simulink model "sampleModel1545"  (R2023a)
settings: Solver=VariableStepAuto  StartTime=0.0  StopTime=10.0  RelTol=1e-3
libraries: hdlsllib x5, simulink x1
settings Model: Creator=user1  LastModifiedBy=user1

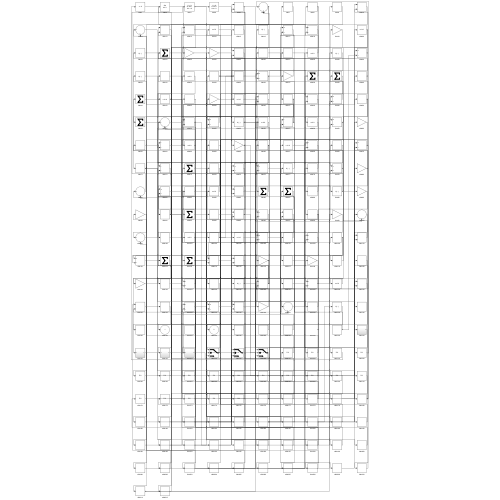
[thumbnail: Simulink's stored preview of the top-level diagram]
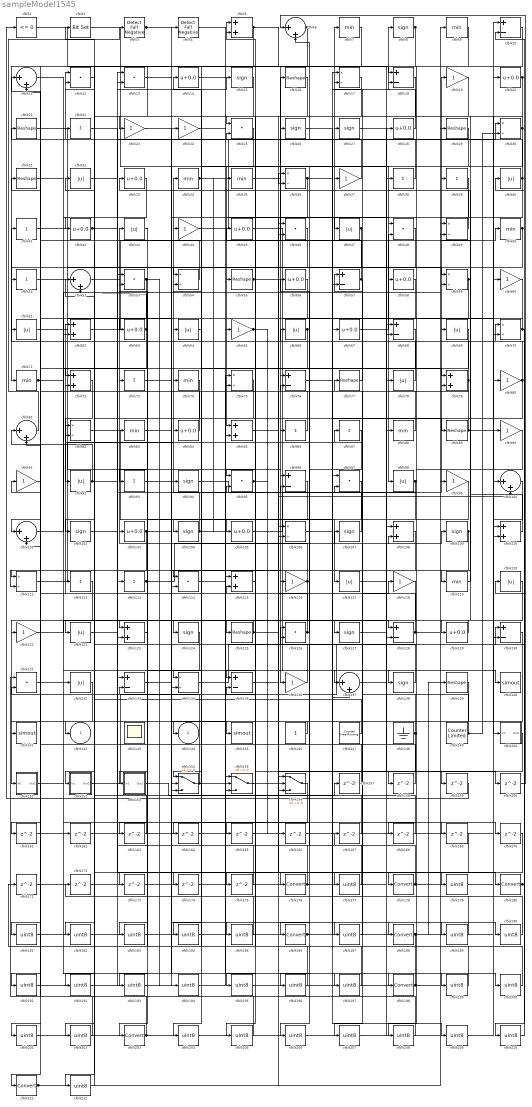
== system sampleModel1545 ==
  cfblk1 : hdlsllib/Logic and Bit Operations/Compare To Zero  relop=<=  OutDataTypeStr=boolean
  cfblk{10,18,57,68,76,96,128,130,133,135} (10 alike) : Sum  Inputs=+-
  cfblk{6,11,52,81,100..101,137} (7 alike) : Sum  Inputs=|++
  cfblk{8,15,26..27,94,102,104,107,109,124,127,138} (12 alike) : Signum
  cfblk{14,20,28,33,42,45,56,58,63,67,84,103,105,129} (14 alike) : Bias  Bias=0.0  SaturateOnIntegerOverflow=off
  cfblk{17,30,36,49,54,59,70,75,82,106,111,134} (12 alike) : Product  Inputs=*/  RndMeth=Zero  SaturateOnIntegerOverflow=on
  cfblk{5,62,72,79,85,108,110,115,123} (9 alike) : Sum
  cfblk{22,38..39,41,51,73,86..87,93,112..113} (11 alike) : Sum  Inputs=+
  cfblk{12..13,25,46,48,53,95,97,114,126,131} (11 alike) : DotProduct  OutDataTypeStr=Inherit: Inherit via internal rule
  cfblk{19,23..24,37,44,60,65,80,90..91,99,116,118,121,136} (15 alike) : Gain
  cfblk{32,40,43,47,61,64,66,69,78,92,98,117,120,122,132} (15 alike) : Abs  SaturateOnIntegerOverflow=off
  cfblk{7,9,34..35,50,71,74,83,88,119} (10 alike) : MinMax
  cfblk{16,21,29,31,55,77,89,125,139} (9 alike) : Reshape
  cfblk140 : ToWorkspace  VariableName=simout  SaveFormat=Timeseries  SampleTime=-1
  cfblk141 : ToWorkspace  VariableName=simout  SaveFormat=Timeseries  SampleTime=-1
  cfblk143 : Scope
      settings: Floating=on
  cfblk145 : ToWorkspace  VariableName=simout  SaveFormat=Timeseries  SampleTime=-1
  cfblk146 : Constant  SampleTime=-1
  cfblk147 : hdlsllib/Sources/Counter Free-Running  NumBits=16  tsamp=-1
  cfblk148 : Ground
  cfblk149 : hdlsllib/Sources/Counter Limited  uplimit=7  tsamp=-1
  cfblk150 : Subsystem
      settings: LibrarySourceBlock=|
      | hdlsllib/Ports &
      | Subsystems/Subsystem
  cfblk151 : Subsystem
      settings: LibrarySourceBlock=|
      | hdlsllib/Ports &
      | Subsystems/Subsystem
  cfblk152 : Subsystem
      settings: LibrarySourceBlock=|
      | hdlsllib/Ports &
      | Subsystems/Subsystem
  cfblk153 : Subsystem
      settings: LibrarySourceBlock=|
      | hdlsllib/Ports &
      | Subsystems/Subsystem
  cfblk154 : Switch  SaturateOnIntegerOverflow=off  InputSameDT=off
  cfblk155 : Switch  SaturateOnIntegerOverflow=off  InputSameDT=off
  cfblk156 : Switch  SaturateOnIntegerOverflow=off  InputSameDT=off
  cfblk{157..175} (19 alike) : Delay  SampleTime=1
  cfblk{176,178,180,186,188,198,203,211} (8 alike) : DataTypeConversion  SaturateOnIntegerOverflow=off  RndMeth=Floor
  cfblk{177,179,181..185,187,189..197,199..202,204..210,212} (29 alike) : DataTypeConversion  OutDataTypeStr=uint8  SaturateOnIntegerOverflow=off  RndMeth=Floor
  cfblk2 : simulink/Logic and Bit Operations/Bit Set  iBit=0
      settings: LibrarySourceBlock=|
      | hdlsllib/Logic and Bit
      | Operations/Bit Set
  cfblk3 : hdlsllib/Logic and Bit Operations/Detect Fall Negative  vinit=0  OutDataTypeStr=boolean
  cfblk4 : hdlsllib/Logic and Bit Operations/Detect Fall Negative  vinit=0  OutDataTypeStr=boolean
  cfblk142 : Outport  VectorParamsAs1DForOutWhenUnconnected=off
  cfblk144 : Outport  Port=2  VectorParamsAs1DForOutWhenUnconnected=off
  wires:
  cfblk98/1 -> cfblk117/1, cfblk97/2
  cfblk104/1 -> cfblk34/1, cfblk108/2, cfblk35/1
  cfblk120/1 -> cfblk151/1(In1)
  cfblk7/1 -> cfblk71/1
  cfblk6/1 -> cfblk136/1, cfblk42/1
  cfblk111/1 -> cfblk84/1
  cfblk40/1 -> cfblk12/1, cfblk154/2
  cfblk79/1 -> cfblk41/1, cfblk76/2
  cfblk116/1 -> cfblk43/1, cfblk154/3, cfblk173/1
  cfblk152/1(Out1) -> cfblk70/1
  cfblk146/1 -> cfblk142/1
  cfblk49/1 -> cfblk33/1
  cfblk2/1 -> cfblk98/1
  cfblk55/1 -> cfblk137/1, cfblk169/1
  cfblk56/1 -> cfblk104/1
  cfblk128/1 -> cfblk77/1, cfblk30/1
  cfblk52/1 -> cfblk7/1
  cfblk90/1 -> cfblk178/1
  cfblk129/1 -> cfblk123/1
  cfblk30/1 -> cfblk25/1, cfblk206/1
  cfblk21/1 -> cfblk96/1
  cfblk44/1 -> cfblk48/1
  cfblk22/1 -> cfblk113/1
  cfblk105/1 -> cfblk19/1
  cfblk25/1 -> cfblk85/1
  cfblk148/1 -> cfblk82/2, cfblk196/1
  cfblk78/1 -> cfblk66/1
  cfblk4/1 -> cfblk65/1
  cfblk135/1 -> cfblk118/1
  cfblk133/1 -> cfblk198/1
  cfblk102/1 -> cfblk27/1
  cfblk32/1 -> cfblk59/1
  cfblk134/1 -> cfblk130/1
  cfblk38/1 -> cfblk21/1
  cfblk81/1 -> cfblk3/1
  cfblk110/1 -> cfblk49/1
  cfblk83/1 -> cfblk145/1
  cfblk11/1 -> cfblk138/1
  cfblk66/1 -> cfblk124/1, cfblk85/2
  cfblk82/1 -> cfblk137/2
  cfblk96/1 -> cfblk105/1
  cfblk67/1 -> cfblk48/2
  cfblk69/1 -> cfblk86/1
  cfblk43/1 -> cfblk93/1
  cfblk95/1 -> cfblk45/1, cfblk166/1
  cfblk126/1 -> cfblk62/1, cfblk56/1, cfblk101/2
  cfblk62/1 -> cfblk16/1
  cfblk84/1 -> cfblk32/1
  cfblk137/1 -> cfblk108/1
  cfblk26/1 -> cfblk89/1
  cfblk72/1 -> cfblk92/1
  cfblk154/1 -> cfblk61/1, cfblk197/1
  cfblk117/1 -> cfblk78/1
  cfblk113/1 -> cfblk107/1, cfblk189/1
  cfblk35/1 -> cfblk26/1
  cfblk73/1 -> cfblk176/1
  cfblk59/1 -> cfblk39/1, cfblk114/1
  cfblk71/1 -> cfblk132/1, cfblk199/1
  cfblk19/1 -> cfblk102/1
  cfblk28/1 -> cfblk8/1
  cfblk70/1 -> cfblk63/1, cfblk210/1
  cfblk99/1 -> cfblk203/1
  cfblk34/1 -> cfblk9/1, cfblk106/1
  cfblk39/1 -> cfblk47/1
  cfblk65/1 -> cfblk135/1, cfblk156/2
  cfblk77/1 -> cfblk37/1
  cfblk20/1 -> cfblk119/1, cfblk110/2
  cfblk92/1 -> cfblk81/1, cfblk95/2, cfblk140/1, cfblk212/1
  cfblk86/1 -> cfblk44/1
  cfblk89/1 -> cfblk60/1, cfblk79/2
  cfblk1/1 -> cfblk88/1
  cfblk48/1 -> cfblk58/1
  cfblk108/1 -> cfblk127/1
  cfblk15/1 -> cfblk152/1(In1)
  cfblk54/1 -> cfblk31/1
  cfblk132/1 -> cfblk141/1
  cfblk149/1 -> cfblk126/1, cfblk30/2
  cfblk8/1 -> cfblk54/1, cfblk181/1
  cfblk60/1 -> cfblk134/1
  cfblk119/1 -> cfblk69/1
  cfblk88/1 -> cfblk11/1
  cfblk17/1 -> cfblk72/1
  cfblk18/1 -> cfblk95/1
  cfblk109/1 -> cfblk134/2, cfblk161/1
  cfblk51/1 -> cfblk94/1
  cfblk3/1 -> cfblk4/1, cfblk79/1
  cfblk80/1 -> cfblk144/1, cfblk57/1
  cfblk61/1 -> cfblk156/1
  cfblk94/1 -> cfblk96/2
  cfblk100/1 -> cfblk130/2
  cfblk14/1 -> cfblk188/1
  cfblk57/1 -> cfblk17/2, cfblk5/1, cfblk5/2, cfblk207/1
  cfblk36/1 -> cfblk18/2, cfblk164/1
  cfblk63/1 -> cfblk101/1, cfblk52/2
  cfblk5/1 -> cfblk23/1, cfblk18/1
  cfblk33/1 -> cfblk62/2
  cfblk87/1 -> cfblk186/1
  cfblk114/1 -> cfblk109/1
  cfblk101/1 -> cfblk59/2
  cfblk31/1 -> cfblk76/1
  cfblk46/1 -> cfblk153/1(In1)
  cfblk103/1 -> cfblk116/1, cfblk111/2
  cfblk41/1 -> cfblk55/1
  cfblk29/1 -> cfblk154/1
  cfblk45/1 -> cfblk150/1(In1)
  cfblk74/1 -> cfblk123/2
  cfblk147/1 -> cfblk2/1
  cfblk107/1 -> cfblk74/1
  cfblk16/1 -> cfblk36/2
  cfblk97/1 -> cfblk125/1
  cfblk37/1 -> cfblk6/2
  cfblk123/1 -> cfblk83/1
  cfblk138/1 -> cfblk53/2
  cfblk155/1 -> cfblk180/1
  cfblk47/1 -> cfblk51/1, cfblk114/2
  cfblk125/1 -> cfblk121/1, cfblk158/1
  cfblk42/1 -> cfblk15/1, cfblk174/1
  cfblk136/1 -> cfblk82/1
  cfblk85/1 -> cfblk100/2
  cfblk12/1 -> cfblk122/1
  cfblk53/1 -> cfblk81/2, cfblk194/1
  cfblk121/1 -> cfblk128/1
  cfblk106/1 -> cfblk50/1
  cfblk112/1 -> cfblk211/1
  cfblk50/1 -> cfblk129/1, cfblk111/1
  cfblk153/1(Out1) -> cfblk157/1
  cfblk157/1 -> cfblk17/1
  cfblk158/1 -> cfblk11/2
  cfblk127/1 -> cfblk159/1
  cfblk159/1 -> cfblk1/1
  cfblk27/1 -> cfblk160/1
  cfblk160/1 -> cfblk6/1
  cfblk161/1 -> cfblk70/2
  cfblk151/1(Out1) -> cfblk162/1
  cfblk162/1 -> cfblk52/1
  cfblk58/1 -> cfblk163/1
  cfblk163/1 -> cfblk12/2
  cfblk164/1 -> cfblk110/1
  cfblk150/1(Out1) -> cfblk165/1
  cfblk165/1 -> cfblk36/1
  cfblk166/1 -> cfblk57/2
  cfblk167/1 -> cfblk72/2
  cfblk9/1 -> cfblk168/1
  cfblk168/1 -> cfblk135/2
  cfblk131/1 -> cfblk170/1
  cfblk171/1 -> cfblk156/3
  cfblk172/1 -> cfblk13/2
  cfblk174/1 -> cfblk128/2
  cfblk23/1 -> cfblk175/1
  cfblk175/1 -> cfblk53/1
  cfblk176/1 -> cfblk97/1, cfblk25/2
  cfblk118/1 -> cfblk177/1
  cfblk177/1 -> cfblk73/1
  cfblk178/1 -> cfblk167/1, cfblk126/2, cfblk20/1
  cfblk122/1 -> cfblk179/1
  cfblk179/1 -> cfblk90/1
  cfblk180/1 -> cfblk40/1, cfblk120/1
  cfblk181/1 -> cfblk155/1
  cfblk170/1 -> cfblk182/1
  cfblk182/1 -> cfblk155/2
  cfblk169/1 -> cfblk183/1
  cfblk183/1 -> cfblk155/3
  cfblk64/1 -> cfblk184/1
  cfblk184/1 -> cfblk80/1
  cfblk13/1 -> cfblk185/1
  cfblk185/1 -> cfblk64/1
  cfblk186/1 -> cfblk67/1, cfblk28/1
  cfblk93/1 -> cfblk187/1
  cfblk187/1 -> cfblk87/1
  cfblk188/1 -> cfblk171/1, cfblk139/1, cfblk100/1
  cfblk189/1 -> cfblk14/1
  cfblk24/1 -> cfblk190/1
  cfblk190/1 -> cfblk172/1
  cfblk139/1 -> cfblk191/1
  cfblk191/1 -> cfblk24/1
  cfblk75/1 -> cfblk192/1
  cfblk192/1 -> cfblk13/1
  cfblk124/1 -> cfblk193/1
  cfblk193/1 -> cfblk75/1
  cfblk194/1 -> cfblk75/2
  cfblk115/1 -> cfblk195/1
  cfblk195/1 -> cfblk49/2
  cfblk196/1 -> cfblk115/1
  cfblk197/1 -> cfblk115/2
  cfblk198/1 -> cfblk54/2, cfblk103/1
  cfblk199/1 -> cfblk133/1
  cfblk173/1 -> cfblk200/1
  cfblk200/1 -> cfblk133/2
  cfblk91/1 -> cfblk201/1
  cfblk201/1 -> cfblk46/1
  cfblk130/1 -> cfblk202/1
  cfblk202/1 -> cfblk91/1
  cfblk203/1 -> cfblk38/1, cfblk46/2, cfblk22/1
  cfblk156/1 -> cfblk204/1
  cfblk204/1 -> cfblk99/1
  cfblk68/1 -> cfblk205/1
  cfblk205/1 -> cfblk131/1
  cfblk206/1 -> cfblk68/1
  cfblk207/1 -> cfblk68/2
  cfblk10/1 -> cfblk208/1
  cfblk208/1 -> cfblk131/2
  cfblk76/1 -> cfblk209/1
  cfblk209/1 -> cfblk10/1
  cfblk210/1 -> cfblk10/2
  cfblk211/1 -> cfblk106/2, cfblk29/1
  cfblk212/1 -> cfblk112/1

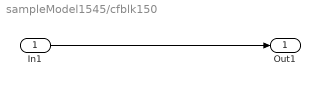
== system sampleModel1545/cfblk150 ==
  In1 : Inport
  Out1 : Outport
  wires:
  In1/1 -> Out1/1

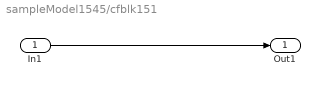
== system sampleModel1545/cfblk151 ==
  In1 : Inport
  Out1 : Outport
  wires:
  In1/1 -> Out1/1

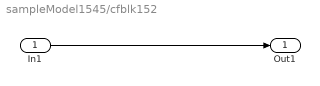
== system sampleModel1545/cfblk152 ==
  In1 : Inport
  Out1 : Outport
  wires:
  In1/1 -> Out1/1

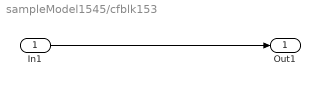
== system sampleModel1545/cfblk153 ==
  In1 : Inport
  Out1 : Outport
  wires:
  In1/1 -> Out1/1
